simulink model "PID_Dual_Robot"  (R2015b)
settings: Solver=ode4  StartTime=0.0  StopTime=10  FixedStep=0.01  RelTol=1e-3
InitFcn:
  | Set_Parameter_line_circle
StopFcn:
  | DrawResult_Dual
values from neighbouring files (symbols this model uses):
  b = 0.1    [Set_Parameter.m]    (also in Set_Parameter_Single.m; Set_Parameter_line_circle.m; Set_Parameter_line_circle_DC_model_no_vision_controller.m; Set_Parameter_sewing_DC_model_no_vision_controller.m)
  D = [30,30,20,20,20,20,20,20]    [Set_Parameter.m]    (also in Set_Parameter_Single.m; Set_Parameter_line_circle.m; Set_Parameter_line_circle_DC_model_no_vision_controller.m; Set_Parameter_line_circle_no_vision_controller.m = [40,40,40,30,20,30,20,20])
  I = [10,10,5,5,5,2,2,2]    [Set_Parameter.m]    (also in Set_Parameter_Single.m; Set_Parameter_line_circle.m; Set_Parameter_line_circle_DC_model_no_vision_controller.m; Set_Parameter_line_circle_no_vision_controller.m = [5,5,5,2,2,2,1,1])
  IniJointAngle_L = theta_L    [Set_Parameter.m]    (also in Set_Parameter_Single.m; Set_Parameter_line_circle.m; Set_Parameter_line_circle_DC_model_no_vision_controller.m; Set_Parameter_line_circle_no_vision_controller.m)
  IniJointAngle_R = theta_R    [Set_Parameter.m]    (also in Set_Parameter_Single.m; Set_Parameter_line_circle.m; Set_Parameter_line_circle_DC_model_no_vision_controller.m; Set_Parameter_line_circle_no_vision_controller.m)
  J = [0.016,0.016,0.012,0.012,0.01,0.01,0.01]    [Set_Parameter.m]    (also in Set_Parameter_Single.m; Set_Parameter_line_circle.m; Set_Parameter_line_circle_DC_model_no_vision_controller.m; Set_Parameter_line_circle_no_vision_controller.m = [10,10,8,8,4,4,4])
  K = 0.01    [Set_Parameter.m]    (also in Set_Parameter_Single.m; Set_Parameter_line_circle.m; Set_Parameter_line_circle_DC_model_no_vision_controller.m; Set_Parameter_sewing_DC_model_no_vision_controller.m)
  L = 0.5    [Set_Parameter.m]    (also in Set_Parameter_Single.m; Set_Parameter_line_circle.m; Set_Parameter_line_circle_DC_model_no_vision_controller.m; Set_Parameter_sewing_DC_model_no_vision_controller.m)
  P = [60,60,50,50,30,30,20,20]    [Set_Parameter.m]    (also in Set_Parameter_Single.m; Set_Parameter_line_circle.m; Set_Parameter_line_circle_DC_model_no_vision_controller.m = [120,120,100,100,60,60,40,40]; Set_Parameter_line_circle_no_vision_controller.m = [350,100,300,150,50,100,20,20])
  R = R_z1x2y3(PoseAngle(1),PoseAngle(2),PoseAngle(3))    [IK_7DOF_FB7roll.m]    (also in Set_Parameter.m = 1; Set_Parameter_Single.m = 1; Set_Parameter_line_circle.m = 1; Set_Parameter_line_circle_DC_model_no_vision_controller.m = 1)
  TOP_D = 0.9    [Set_Parameter.m]    (also in Set_Parameter_Single.m; Set_Parameter_line_circle.m; Set_Parameter_sewing_DC_model_no_vision_controller.m)
  TOP_I = 1    [Set_Parameter.m]    (also in Set_Parameter_Single.m; Set_Parameter_line_circle.m; Set_Parameter_sewing_DC_model_no_vision_controller.m)
  TOP_P = 5    [Set_Parameter.m]    (also in Set_Parameter_Single.m; Set_Parameter_line_circle.m; Set_Parameter_sewing_DC_model_no_vision_controller.m)
libraries: simulink x14
settings Model: Creator=User  LastModifiedBy=User

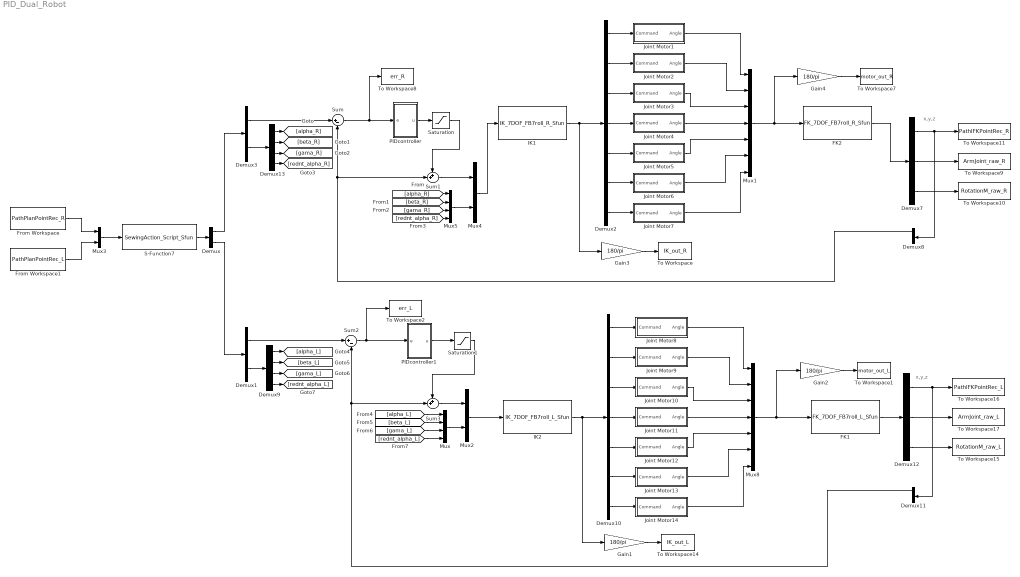
== system PID_Dual_Robot ==
  note: x,y,z
  note: x,y,z
  Demux : Demux  Outputs=[7,7]
  Demux{1,3,8,11} (4 alike) : Demux  Outputs=[3,4]
  Demux10 : Demux  Outputs=7
  Demux12 : Demux  Outputs=[7,30,9]
  Demux13 : Demux
  Demux2 : Demux  Outputs=7
  Demux7 : Demux  Outputs=[7,30,9]
  Demux9 : Demux
  FK1 : S-Function  FunctionName=FK_7DOF_FB7roll_L_Sfun  SFunctionDeploymentMode=off  EnableBusSupport=off
  FK2 : S-Function  FunctionName=FK_7DOF_FB7roll_R_Sfun  SFunctionDeploymentMode=off  EnableBusSupport=off
  From Workspace : FromWorkspace  VariableName=PathPlanPointRec_R  SampleTime=0
  From Workspace1 : FromWorkspace  VariableName=PathPlanPointRec_L  SampleTime=0
  Gain{1..4} (4 alike) : Gain  Gain=180/pi
  IK1 : S-Function  FunctionName=IK_7DOF_FB7roll_R_Sfun  SFunctionDeploymentMode=off  EnableBusSupport=off
  IK2 : S-Function  FunctionName=IK_7DOF_FB7roll_L_Sfun  SFunctionDeploymentMode=off  EnableBusSupport=off
  Joint Motor1 : Subsystem
  Joint Motor10 : Subsystem
  Joint Motor11 : Subsystem
  Joint Motor12 : Subsystem
  Joint Motor13 : Subsystem
  Joint Motor14 : Subsystem
  Joint Motor2 : Subsystem
  Joint Motor3 : Subsystem
  Joint Motor4 : Subsystem
  Joint Motor5 : Subsystem
  Joint Motor6 : Subsystem
  Joint Motor7 : Subsystem
  Joint Motor8 : Subsystem
  Joint Motor9 : Subsystem
  Mux : Mux
  Mux1 : Mux  Inputs=7
  Mux2 : Mux  Inputs=[3,4]
  Mux3 : Mux  Inputs=[7,7]
  Mux4 : Mux  Inputs=[3,4]
  Mux5 : Mux
  Mux8 : Mux  Inputs=7
  PIDcontroller : Subsystem
  PIDcontroller1 : Subsystem
  S-Function7 : S-Function  FunctionName=SewingAction_Script_Sfun  SFunctionDeploymentMode=off  EnableBusSupport=off
  Saturation : Saturate  UpperLimit=50  LowerLimit=-50
  Saturation1 : Saturate  UpperLimit=50  LowerLimit=-50
  Sum : Sum  Inputs=|+-
  Sum1 : Sum  Inputs=++|
  Sum2 : Sum  Inputs=|+-
  Sum3 : Sum  Inputs=++|
  To Workspace : ToWorkspace  VariableName=IK_out_R  SaveFormat=Timeseries  SampleTime=-1
  To Workspace1 : ToWorkspace  VariableName=motor_out_L  SaveFormat=Timeseries  SampleTime=-1
  To Workspace10 : ToWorkspace  VariableName=RotationM_raw_R  SaveFormat=Timeseries  SampleTime=-1
  To Workspace11 : ToWorkspace  VariableName=PathIFKPointRec_R  SaveFormat=Timeseries  SampleTime=-1
  To Workspace14 : ToWorkspace  VariableName=IK_out_L  SaveFormat=Timeseries  SampleTime=-1
  To Workspace15 : ToWorkspace  VariableName=RotationM_raw_L  SaveFormat=Timeseries  SampleTime=-1
  To Workspace16 : ToWorkspace  VariableName=PathIFKPointRec_L  SaveFormat=Timeseries  SampleTime=-1
  To Workspace17 : ToWorkspace  VariableName=ArmJoint_raw_L  SaveFormat=Timeseries  SampleTime=-1
  To Workspace2 : ToWorkspace  VariableName=err_L  SaveFormat=Timeseries  SampleTime=-1
  To Workspace7 : ToWorkspace  VariableName=motor_out_R  SaveFormat=Timeseries  SampleTime=-1
  To Workspace8 : ToWorkspace  VariableName=err_R  SaveFormat=Timeseries  SampleTime=-1
  To Workspace9 : ToWorkspace  VariableName=ArmJoint_raw_R  SaveFormat=Timeseries  SampleTime=-1
  wires:
  Joint Motor3/1(Angle) -> Mux1/3
  Joint Motor1/1(Angle) -> Mux1/1
  Joint Motor2/1(Angle) -> Mux1/2
  Joint Motor4/1(Angle) -> Mux1/4
  Joint Motor5/1(Angle) -> Mux1/5
  Joint Motor6/1(Angle) -> Mux1/6
  Joint Motor7/1(Angle) -> Mux1/7
  Gain3/1 -> To Workspace/1
  Gain4/1 -> To Workspace7/1
  Demux2/6 -> Joint Motor6/1(Command)
  Demux2/5 -> Joint Motor5/1(Command)
  Demux2/4 -> Joint Motor4/1(Command)
  Demux2/1 -> Joint Motor1/1(Command)
  Demux2/2 -> Joint Motor2/1(Command)
  Demux2/3 -> Joint Motor3/1(Command)
  IK1/1 -> Demux2/1, Gain3/1
  Mux1/1 -> Gain4/1, FK2/1
  Sum/1 -> PIDcontroller/1(e), To Workspace8/1
  Mux4/1 -> IK1/1
  PIDcontroller/1(u) -> Saturation/1
  Saturation/1 -> Sum1/1
  FK2/1 -> Demux7/1
  Demux7/1 -> To Workspace11/1, Demux8/1
  Demux7/2 -> To Workspace9/1
  Demux7/3 -> To Workspace10/1
  Demux8/1 -> Sum/2, Sum1/2
  S-Function7/1 -> Demux/1
  Demux/1 -> Demux3/1
  Demux/2 -> Demux1/1
  Sum2/1 -> To Workspace2/1, PIDcontroller1/1(e)
  PIDcontroller1/1(u) -> Saturation1/1
  Saturation1/1 -> Sum3/1
  Demux9/1 -> [alpha_L]
  Demux9/2 -> [beta_L]
  Demux9/3 -> [gama_L]
  Demux9/4 -> [rednt_alpha_L]
  Demux1/2 -> Demux9/1
  [alpha_L] -> Mux/1
  [beta_L] -> Mux/2
  [gama_L] -> Mux/3
  [rednt_alpha_L] -> Mux/4
  Mux/1 -> Mux2/2
  Joint Motor10/1(Angle) -> Mux8/3
  Joint Motor8/1(Angle) -> Mux8/1
  Joint Motor9/1(Angle) -> Mux8/2
  Joint Motor11/1(Angle) -> Mux8/4
  Joint Motor12/1(Angle) -> Mux8/5
  Joint Motor13/1(Angle) -> Mux8/6
  Joint Motor14/1(Angle) -> Mux8/7
  Demux10/7 -> Joint Motor14/1(Command)
  Demux10/6 -> Joint Motor13/1(Command)
  Demux10/5 -> Joint Motor12/1(Command)
  Demux10/4 -> Joint Motor11/1(Command)
  Demux10/1 -> Joint Motor8/1(Command)
  Demux10/2 -> Joint Motor9/1(Command)
  Demux10/3 -> Joint Motor10/1(Command)
  Gain1/1 -> To Workspace14/1
  IK2/1 -> Demux10/1, Gain1/1
  FK1/1 -> Demux12/1
  Demux12/2 -> To Workspace17/1
  Demux12/1 -> To Workspace16/1, Demux11/1
  Demux12/3 -> To Workspace15/1
  Demux3/1 -> Sum/1
  Demux3/2 -> Demux13/1
  Demux13/2 -> [beta_R]
  Demux13/3 -> [gama_R]
  Demux13/4 -> [rednt_alpha_R]
  Gain2/1 -> To Workspace1/1
  Mux8/1 -> FK1/1, Gain2/1
  Mux3/1 -> S-Function7/1
  From Workspace/1 -> Mux3/1
  From Workspace1/1 -> Mux3/2
  Mux2/1 -> IK2/1
  Demux1/1 -> Sum2/1
  Sum3/1 -> Mux2/1
  Demux11/1 -> Sum3/2, Sum2/2
  Sum1/1 -> Mux4/1
  Mux5/1 -> Mux4/2
  [alpha_R] -> Mux5/1
  [beta_R] -> Mux5/2
  [gama_R] -> Mux5/3
  [rednt_alpha_R] -> Mux5/4
  Demux2/7 -> Joint Motor7/1(Command)
  Demux13/1 -> [alpha_R]

== system PID_Dual_Robot/Joint Motor1 ==
  Command : Inport
  Constant : Constant  Value=IniJointAngle_R(1)
  DC motor : Subsystem
  Gain : Gain  Gain=2
  Integrator : Integrator  InitialConditionSource=external
  PID Controller : simulink/Continuous/PID Controller  Controller=PID  TimeDomain=Continuous-time  SampleTime=-1  IntegratorMethod=Forward Euler  FilterMethod=Forward Euler  Form=Parallel  UseFilter=on  ControllerParametersSource=internal  P=P(1)  I=I(1)  D=D(1)  N=0  InitialConditionSource=internal  InitialConditionForIntegrator=0  InitialConditionForFilter=0  ExternalReset=none  LimitOutput=off  UpperSaturationLimit=inf  LowerSaturationLimit=-inf  LinearizeAsGain=on  AntiWindupMode=none  Kb=1  TrackingMode=off  Kt=1  PParamMin=[]  PParamMax=[]  IParamMin=[]  IParamMax=[]  DParamMin=[]  DParamMax=[]  NParamMin=[]  NParamMax=[]  KbParamMin=[]  KbParamMax=[]  KtParamMin=[]  KtParamMax=[]  POutMin=[]  POutMax=[]  IOutMin=[]  IOutMax=[]  DOutMin=[]  DOutMax=[]  NOutMin=[]  NOutMax=[]  KbOutMin=[]  KbOutMax=[]  KtOutMin=[]  KtOutMax=[]  IntegratorOutMin=[]  IntegratorOutMax=[]  FilterOutMin=[]  FilterOutMax=[]  SumOutMin=[]  SumOutMax=[]  SumI1OutMin=[]  SumI1OutMax=[]  SumI2OutMin=[]  SumI2OutMax=[]  SumI3OutMin=[]  SumI3OutMax=[]  SumDOutMin=[]  SumDOutMax=[]  SaturationOutMin=[]  SaturationOutMax=[]  IntegratorContinuousStateAttributes=''  IntegratorStateMustResolveToSignalObject=off  IntegratorRTWStateStorageClass=Auto  FilterContinuousStateAttributes=''  FilterStateMustResolveToSignalObject=off  FilterRTWStateStorageClass=Auto  DifferentiatorICPrevScaledInput=0  DifferentiatorOutMin=[]  DifferentiatorOutMax=[]
  Sum : Sum  Inputs=|+-
  Sum1 : Sum  Inputs=|+-
  Angle : Outport
  wires:
  Sum/1 -> PID Controller/1
  PID Controller/1 -> DC motor/1(Voltage)
  DC motor/1(Speed) -> Sum/2, Integrator/1
  Integrator/1 -> Angle/1, Sum1/2
  Command/1 -> Sum1/1
  Sum1/1 -> Gain/1
  Gain/1 -> Sum/1
  Constant/1 -> Integrator/2

== system PID_Dual_Robot/Joint Motor10 ==
  Command : Inport
  Constant : Constant  Value=IniJointAngle_L(3)
  DC motor : Subsystem
  Gain : Gain  Gain=2
  Integrator : Integrator  InitialConditionSource=external
  PID Controller : simulink/Continuous/PID Controller  Controller=PID  TimeDomain=Continuous-time  SampleTime=-1  IntegratorMethod=Forward Euler  FilterMethod=Forward Euler  Form=Parallel  UseFilter=on  ControllerParametersSource=internal  P=P(3)  I=I(3)  D=D(3)  N=0  InitialConditionSource=internal  InitialConditionForIntegrator=0  InitialConditionForFilter=0  ExternalReset=none  LimitOutput=off  UpperSaturationLimit=inf  LowerSaturationLimit=-inf  LinearizeAsGain=on  AntiWindupMode=none  Kb=1  TrackingMode=off  Kt=1  PParamMin=[]  PParamMax=[]  IParamMin=[]  IParamMax=[]  DParamMin=[]  DParamMax=[]  NParamMin=[]  NParamMax=[]  KbParamMin=[]  KbParamMax=[]  KtParamMin=[]  KtParamMax=[]  POutMin=[]  POutMax=[]  IOutMin=[]  IOutMax=[]  DOutMin=[]  DOutMax=[]  NOutMin=[]  NOutMax=[]  KbOutMin=[]  KbOutMax=[]  KtOutMin=[]  KtOutMax=[]  IntegratorOutMin=[]  IntegratorOutMax=[]  FilterOutMin=[]  FilterOutMax=[]  SumOutMin=[]  SumOutMax=[]  SumI1OutMin=[]  SumI1OutMax=[]  SumI2OutMin=[]  SumI2OutMax=[]  SumI3OutMin=[]  SumI3OutMax=[]  SumDOutMin=[]  SumDOutMax=[]  SaturationOutMin=[]  SaturationOutMax=[]  IntegratorContinuousStateAttributes=''  IntegratorStateMustResolveToSignalObject=off  IntegratorRTWStateStorageClass=Auto  FilterContinuousStateAttributes=''  FilterStateMustResolveToSignalObject=off  FilterRTWStateStorageClass=Auto  DifferentiatorICPrevScaledInput=0  DifferentiatorOutMin=[]  DifferentiatorOutMax=[]
  Sum : Sum  Inputs=|+-
  Sum1 : Sum  Inputs=|+-
  Angle : Outport
  wires:
  Sum/1 -> PID Controller/1
  PID Controller/1 -> DC motor/1(Voltage)
  DC motor/1(Speed) -> Sum/2, Integrator/1
  Integrator/1 -> Angle/1, Sum1/2
  Command/1 -> Sum1/1
  Sum1/1 -> Gain/1
  Gain/1 -> Sum/1
  Constant/1 -> Integrator/2

== system PID_Dual_Robot/Joint Motor11 ==
  Command : Inport
  Constant : Constant  Value=IniJointAngle_L(4)
  DC motor : Subsystem
  Gain : Gain  Gain=2
  Integrator : Integrator  InitialConditionSource=external
  PID Controller : simulink/Continuous/PID Controller  Controller=PID  TimeDomain=Continuous-time  SampleTime=-1  IntegratorMethod=Forward Euler  FilterMethod=Forward Euler  Form=Parallel  UseFilter=on  ControllerParametersSource=internal  P=P(4)  I=I(4)  D=D(4)  N=0  InitialConditionSource=internal  InitialConditionForIntegrator=0  InitialConditionForFilter=0  ExternalReset=none  LimitOutput=off  UpperSaturationLimit=inf  LowerSaturationLimit=-inf  LinearizeAsGain=on  AntiWindupMode=none  Kb=1  TrackingMode=off  Kt=1  PParamMin=[]  PParamMax=[]  IParamMin=[]  IParamMax=[]  DParamMin=[]  DParamMax=[]  NParamMin=[]  NParamMax=[]  KbParamMin=[]  KbParamMax=[]  KtParamMin=[]  KtParamMax=[]  POutMin=[]  POutMax=[]  IOutMin=[]  IOutMax=[]  DOutMin=[]  DOutMax=[]  NOutMin=[]  NOutMax=[]  KbOutMin=[]  KbOutMax=[]  KtOutMin=[]  KtOutMax=[]  IntegratorOutMin=[]  IntegratorOutMax=[]  FilterOutMin=[]  FilterOutMax=[]  SumOutMin=[]  SumOutMax=[]  SumI1OutMin=[]  SumI1OutMax=[]  SumI2OutMin=[]  SumI2OutMax=[]  SumI3OutMin=[]  SumI3OutMax=[]  SumDOutMin=[]  SumDOutMax=[]  SaturationOutMin=[]  SaturationOutMax=[]  IntegratorContinuousStateAttributes=''  IntegratorStateMustResolveToSignalObject=off  IntegratorRTWStateStorageClass=Auto  FilterContinuousStateAttributes=''  FilterStateMustResolveToSignalObject=off  FilterRTWStateStorageClass=Auto  DifferentiatorICPrevScaledInput=0  DifferentiatorOutMin=[]  DifferentiatorOutMax=[]
  Sum : Sum  Inputs=|+-
  Sum1 : Sum  Inputs=|+-
  Angle : Outport
  wires:
  Sum/1 -> PID Controller/1
  PID Controller/1 -> DC motor/1(Voltage)
  DC motor/1(Speed) -> Sum/2, Integrator/1
  Integrator/1 -> Angle/1, Sum1/2
  Command/1 -> Sum1/1
  Sum1/1 -> Gain/1
  Gain/1 -> Sum/1
  Constant/1 -> Integrator/2

== system PID_Dual_Robot/Joint Motor12 ==
  Command : Inport
  Constant : Constant  Value=IniJointAngle_L(5)
  DC motor : Subsystem
  Gain : Gain  Gain=2
  Integrator : Integrator  InitialConditionSource=external
  PID Controller : simulink/Continuous/PID Controller  Controller=PID  TimeDomain=Continuous-time  SampleTime=-1  IntegratorMethod=Forward Euler  FilterMethod=Forward Euler  Form=Parallel  UseFilter=on  ControllerParametersSource=internal  P=P(5)  I=I(5)  D=D(5)  N=0  InitialConditionSource=internal  InitialConditionForIntegrator=0  InitialConditionForFilter=0  ExternalReset=none  LimitOutput=off  UpperSaturationLimit=inf  LowerSaturationLimit=-inf  LinearizeAsGain=on  AntiWindupMode=none  Kb=1  TrackingMode=off  Kt=1  PParamMin=[]  PParamMax=[]  IParamMin=[]  IParamMax=[]  DParamMin=[]  DParamMax=[]  NParamMin=[]  NParamMax=[]  KbParamMin=[]  KbParamMax=[]  KtParamMin=[]  KtParamMax=[]  POutMin=[]  POutMax=[]  IOutMin=[]  IOutMax=[]  DOutMin=[]  DOutMax=[]  NOutMin=[]  NOutMax=[]  KbOutMin=[]  KbOutMax=[]  KtOutMin=[]  KtOutMax=[]  IntegratorOutMin=[]  IntegratorOutMax=[]  FilterOutMin=[]  FilterOutMax=[]  SumOutMin=[]  SumOutMax=[]  SumI1OutMin=[]  SumI1OutMax=[]  SumI2OutMin=[]  SumI2OutMax=[]  SumI3OutMin=[]  SumI3OutMax=[]  SumDOutMin=[]  SumDOutMax=[]  SaturationOutMin=[]  SaturationOutMax=[]  IntegratorContinuousStateAttributes=''  IntegratorStateMustResolveToSignalObject=off  IntegratorRTWStateStorageClass=Auto  FilterContinuousStateAttributes=''  FilterStateMustResolveToSignalObject=off  FilterRTWStateStorageClass=Auto  DifferentiatorICPrevScaledInput=0  DifferentiatorOutMin=[]  DifferentiatorOutMax=[]
  Sum : Sum  Inputs=|+-
  Sum1 : Sum  Inputs=|+-
  Angle : Outport
  wires:
  Sum/1 -> PID Controller/1
  PID Controller/1 -> DC motor/1(Voltage)
  DC motor/1(Speed) -> Sum/2, Integrator/1
  Integrator/1 -> Angle/1, Sum1/2
  Command/1 -> Sum1/1
  Sum1/1 -> Gain/1
  Gain/1 -> Sum/1
  Constant/1 -> Integrator/2

== system PID_Dual_Robot/Joint Motor13 ==
  Command : Inport
  Constant : Constant  Value=IniJointAngle_L(6)
  DC motor : Subsystem
  Gain : Gain  Gain=2
  Integrator : Integrator  InitialConditionSource=external
  PID Controller : simulink/Continuous/PID Controller  Controller=PID  TimeDomain=Continuous-time  SampleTime=-1  IntegratorMethod=Forward Euler  FilterMethod=Forward Euler  Form=Parallel  UseFilter=on  ControllerParametersSource=internal  P=P(6)  I=I(6)  D=D(6)  N=0  InitialConditionSource=internal  InitialConditionForIntegrator=0  InitialConditionForFilter=0  ExternalReset=none  LimitOutput=off  UpperSaturationLimit=inf  LowerSaturationLimit=-inf  LinearizeAsGain=on  AntiWindupMode=none  Kb=1  TrackingMode=off  Kt=1  PParamMin=[]  PParamMax=[]  IParamMin=[]  IParamMax=[]  DParamMin=[]  DParamMax=[]  NParamMin=[]  NParamMax=[]  KbParamMin=[]  KbParamMax=[]  KtParamMin=[]  KtParamMax=[]  POutMin=[]  POutMax=[]  IOutMin=[]  IOutMax=[]  DOutMin=[]  DOutMax=[]  NOutMin=[]  NOutMax=[]  KbOutMin=[]  KbOutMax=[]  KtOutMin=[]  KtOutMax=[]  IntegratorOutMin=[]  IntegratorOutMax=[]  FilterOutMin=[]  FilterOutMax=[]  SumOutMin=[]  SumOutMax=[]  SumI1OutMin=[]  SumI1OutMax=[]  SumI2OutMin=[]  SumI2OutMax=[]  SumI3OutMin=[]  SumI3OutMax=[]  SumDOutMin=[]  SumDOutMax=[]  SaturationOutMin=[]  SaturationOutMax=[]  IntegratorContinuousStateAttributes=''  IntegratorStateMustResolveToSignalObject=off  IntegratorRTWStateStorageClass=Auto  FilterContinuousStateAttributes=''  FilterStateMustResolveToSignalObject=off  FilterRTWStateStorageClass=Auto  DifferentiatorICPrevScaledInput=0  DifferentiatorOutMin=[]  DifferentiatorOutMax=[]
  Sum : Sum  Inputs=|+-
  Sum1 : Sum  Inputs=|+-
  Angle : Outport
  wires:
  Sum/1 -> PID Controller/1
  PID Controller/1 -> DC motor/1(Voltage)
  DC motor/1(Speed) -> Sum/2, Integrator/1
  Integrator/1 -> Angle/1, Sum1/2
  Command/1 -> Sum1/1
  Sum1/1 -> Gain/1
  Gain/1 -> Sum/1
  Constant/1 -> Integrator/2

== system PID_Dual_Robot/Joint Motor14 ==
  Command : Inport
  Constant : Constant  Value=IniJointAngle_L(7)
  DC motor : Subsystem
  Gain : Gain  Gain=2
  Integrator : Integrator  InitialConditionSource=external
  PID Controller : simulink/Continuous/PID Controller  Controller=PID  TimeDomain=Continuous-time  SampleTime=-1  IntegratorMethod=Forward Euler  FilterMethod=Forward Euler  Form=Parallel  UseFilter=on  ControllerParametersSource=internal  P=P(7)  I=I(7)  D=D(7)  N=0  InitialConditionSource=internal  InitialConditionForIntegrator=0  InitialConditionForFilter=0  ExternalReset=none  LimitOutput=off  UpperSaturationLimit=inf  LowerSaturationLimit=-inf  LinearizeAsGain=on  AntiWindupMode=none  Kb=1  TrackingMode=off  Kt=1  PParamMin=[]  PParamMax=[]  IParamMin=[]  IParamMax=[]  DParamMin=[]  DParamMax=[]  NParamMin=[]  NParamMax=[]  KbParamMin=[]  KbParamMax=[]  KtParamMin=[]  KtParamMax=[]  POutMin=[]  POutMax=[]  IOutMin=[]  IOutMax=[]  DOutMin=[]  DOutMax=[]  NOutMin=[]  NOutMax=[]  KbOutMin=[]  KbOutMax=[]  KtOutMin=[]  KtOutMax=[]  IntegratorOutMin=[]  IntegratorOutMax=[]  FilterOutMin=[]  FilterOutMax=[]  SumOutMin=[]  SumOutMax=[]  SumI1OutMin=[]  SumI1OutMax=[]  SumI2OutMin=[]  SumI2OutMax=[]  SumI3OutMin=[]  SumI3OutMax=[]  SumDOutMin=[]  SumDOutMax=[]  SaturationOutMin=[]  SaturationOutMax=[]  IntegratorContinuousStateAttributes=''  IntegratorStateMustResolveToSignalObject=off  IntegratorRTWStateStorageClass=Auto  FilterContinuousStateAttributes=''  FilterStateMustResolveToSignalObject=off  FilterRTWStateStorageClass=Auto  DifferentiatorICPrevScaledInput=0  DifferentiatorOutMin=[]  DifferentiatorOutMax=[]
  Sum : Sum  Inputs=|+-
  Sum1 : Sum  Inputs=|+-
  Angle : Outport
  wires:
  Sum/1 -> PID Controller/1
  PID Controller/1 -> DC motor/1(Voltage)
  DC motor/1(Speed) -> Sum/2, Integrator/1
  Integrator/1 -> Angle/1, Sum1/2
  Command/1 -> Sum1/1
  Sum1/1 -> Gain/1
  Gain/1 -> Sum/1
  Constant/1 -> Integrator/2

== system PID_Dual_Robot/Joint Motor2 ==
  Command : Inport
  Constant : Constant  Value=IniJointAngle_R(2)
  DC motor : Subsystem
  Gain : Gain  Gain=2
  Integrator : Integrator  InitialConditionSource=external
  PID Controller : simulink/Continuous/PID Controller  Controller=PID  TimeDomain=Continuous-time  SampleTime=-1  IntegratorMethod=Forward Euler  FilterMethod=Forward Euler  Form=Parallel  UseFilter=on  ControllerParametersSource=internal  P=P(2)  I=I(2)  D=D(2)  N=0  InitialConditionSource=internal  InitialConditionForIntegrator=0  InitialConditionForFilter=0  ExternalReset=none  LimitOutput=off  UpperSaturationLimit=inf  LowerSaturationLimit=-inf  LinearizeAsGain=on  AntiWindupMode=none  Kb=1  TrackingMode=off  Kt=1  PParamMin=[]  PParamMax=[]  IParamMin=[]  IParamMax=[]  DParamMin=[]  DParamMax=[]  NParamMin=[]  NParamMax=[]  KbParamMin=[]  KbParamMax=[]  KtParamMin=[]  KtParamMax=[]  POutMin=[]  POutMax=[]  IOutMin=[]  IOutMax=[]  DOutMin=[]  DOutMax=[]  NOutMin=[]  NOutMax=[]  KbOutMin=[]  KbOutMax=[]  KtOutMin=[]  KtOutMax=[]  IntegratorOutMin=[]  IntegratorOutMax=[]  FilterOutMin=[]  FilterOutMax=[]  SumOutMin=[]  SumOutMax=[]  SumI1OutMin=[]  SumI1OutMax=[]  SumI2OutMin=[]  SumI2OutMax=[]  SumI3OutMin=[]  SumI3OutMax=[]  SumDOutMin=[]  SumDOutMax=[]  SaturationOutMin=[]  SaturationOutMax=[]  IntegratorContinuousStateAttributes=''  IntegratorStateMustResolveToSignalObject=off  IntegratorRTWStateStorageClass=Auto  FilterContinuousStateAttributes=''  FilterStateMustResolveToSignalObject=off  FilterRTWStateStorageClass=Auto  DifferentiatorICPrevScaledInput=0  DifferentiatorOutMin=[]  DifferentiatorOutMax=[]
  Sum : Sum  Inputs=|+-
  Sum1 : Sum  Inputs=|+-
  Angle : Outport
  wires:
  Sum/1 -> PID Controller/1
  PID Controller/1 -> DC motor/1(Voltage)
  DC motor/1(Speed) -> Sum/2, Integrator/1
  Integrator/1 -> Angle/1, Sum1/2
  Command/1 -> Sum1/1
  Sum1/1 -> Gain/1
  Gain/1 -> Sum/1
  Constant/1 -> Integrator/2

== system PID_Dual_Robot/Joint Motor3 ==
  Command : Inport
  Constant : Constant  Value=IniJointAngle_R(3)
  DC motor : Subsystem
  Gain : Gain  Gain=2
  Integrator : Integrator  InitialConditionSource=external
  PID Controller : simulink/Continuous/PID Controller  Controller=PID  TimeDomain=Continuous-time  SampleTime=-1  IntegratorMethod=Forward Euler  FilterMethod=Forward Euler  Form=Parallel  UseFilter=on  ControllerParametersSource=internal  P=P(3)  I=I(3)  D=D(3)  N=0  InitialConditionSource=internal  InitialConditionForIntegrator=0  InitialConditionForFilter=0  ExternalReset=none  LimitOutput=off  UpperSaturationLimit=inf  LowerSaturationLimit=-inf  LinearizeAsGain=on  AntiWindupMode=none  Kb=1  TrackingMode=off  Kt=1  PParamMin=[]  PParamMax=[]  IParamMin=[]  IParamMax=[]  DParamMin=[]  DParamMax=[]  NParamMin=[]  NParamMax=[]  KbParamMin=[]  KbParamMax=[]  KtParamMin=[]  KtParamMax=[]  POutMin=[]  POutMax=[]  IOutMin=[]  IOutMax=[]  DOutMin=[]  DOutMax=[]  NOutMin=[]  NOutMax=[]  KbOutMin=[]  KbOutMax=[]  KtOutMin=[]  KtOutMax=[]  IntegratorOutMin=[]  IntegratorOutMax=[]  FilterOutMin=[]  FilterOutMax=[]  SumOutMin=[]  SumOutMax=[]  SumI1OutMin=[]  SumI1OutMax=[]  SumI2OutMin=[]  SumI2OutMax=[]  SumI3OutMin=[]  SumI3OutMax=[]  SumDOutMin=[]  SumDOutMax=[]  SaturationOutMin=[]  SaturationOutMax=[]  IntegratorContinuousStateAttributes=''  IntegratorStateMustResolveToSignalObject=off  IntegratorRTWStateStorageClass=Auto  FilterContinuousStateAttributes=''  FilterStateMustResolveToSignalObject=off  FilterRTWStateStorageClass=Auto  DifferentiatorICPrevScaledInput=0  DifferentiatorOutMin=[]  DifferentiatorOutMax=[]
  Sum : Sum  Inputs=|+-
  Sum1 : Sum  Inputs=|+-
  Angle : Outport
  wires:
  Sum/1 -> PID Controller/1
  PID Controller/1 -> DC motor/1(Voltage)
  DC motor/1(Speed) -> Sum/2, Integrator/1
  Integrator/1 -> Angle/1, Sum1/2
  Command/1 -> Sum1/1
  Sum1/1 -> Gain/1
  Gain/1 -> Sum/1
  Constant/1 -> Integrator/2

== system PID_Dual_Robot/Joint Motor4 ==
  Command : Inport
  Constant : Constant  Value=IniJointAngle_R(4)
  DC motor : Subsystem
  Gain : Gain  Gain=2
  Integrator : Integrator  InitialConditionSource=external
  PID Controller : simulink/Continuous/PID Controller  Controller=PID  TimeDomain=Continuous-time  SampleTime=-1  IntegratorMethod=Forward Euler  FilterMethod=Forward Euler  Form=Parallel  UseFilter=on  ControllerParametersSource=internal  P=P(4)  I=I(4)  D=D(4)  N=0  InitialConditionSource=internal  InitialConditionForIntegrator=0  InitialConditionForFilter=0  ExternalReset=none  LimitOutput=off  UpperSaturationLimit=inf  LowerSaturationLimit=-inf  LinearizeAsGain=on  AntiWindupMode=none  Kb=1  TrackingMode=off  Kt=1  PParamMin=[]  PParamMax=[]  IParamMin=[]  IParamMax=[]  DParamMin=[]  DParamMax=[]  NParamMin=[]  NParamMax=[]  KbParamMin=[]  KbParamMax=[]  KtParamMin=[]  KtParamMax=[]  POutMin=[]  POutMax=[]  IOutMin=[]  IOutMax=[]  DOutMin=[]  DOutMax=[]  NOutMin=[]  NOutMax=[]  KbOutMin=[]  KbOutMax=[]  KtOutMin=[]  KtOutMax=[]  IntegratorOutMin=[]  IntegratorOutMax=[]  FilterOutMin=[]  FilterOutMax=[]  SumOutMin=[]  SumOutMax=[]  SumI1OutMin=[]  SumI1OutMax=[]  SumI2OutMin=[]  SumI2OutMax=[]  SumI3OutMin=[]  SumI3OutMax=[]  SumDOutMin=[]  SumDOutMax=[]  SaturationOutMin=[]  SaturationOutMax=[]  IntegratorContinuousStateAttributes=''  IntegratorStateMustResolveToSignalObject=off  IntegratorRTWStateStorageClass=Auto  FilterContinuousStateAttributes=''  FilterStateMustResolveToSignalObject=off  FilterRTWStateStorageClass=Auto  DifferentiatorICPrevScaledInput=0  DifferentiatorOutMin=[]  DifferentiatorOutMax=[]
  Sum : Sum  Inputs=|+-
  Sum1 : Sum  Inputs=|+-
  Angle : Outport
  wires:
  Sum/1 -> PID Controller/1
  PID Controller/1 -> DC motor/1(Voltage)
  DC motor/1(Speed) -> Sum/2, Integrator/1
  Integrator/1 -> Angle/1, Sum1/2
  Command/1 -> Sum1/1
  Sum1/1 -> Gain/1
  Gain/1 -> Sum/1
  Constant/1 -> Integrator/2

== system PID_Dual_Robot/Joint Motor5 ==
  Command : Inport
  Constant : Constant  Value=IniJointAngle_R(5)
  DC motor : Subsystem
  Gain : Gain  Gain=2
  Integrator : Integrator  InitialConditionSource=external
  PID Controller : simulink/Continuous/PID Controller  Controller=PID  TimeDomain=Continuous-time  SampleTime=-1  IntegratorMethod=Forward Euler  FilterMethod=Forward Euler  Form=Parallel  UseFilter=on  ControllerParametersSource=internal  P=P(5)  I=I(5)  D=D(5)  N=0  InitialConditionSource=internal  InitialConditionForIntegrator=0  InitialConditionForFilter=0  ExternalReset=none  LimitOutput=off  UpperSaturationLimit=inf  LowerSaturationLimit=-inf  LinearizeAsGain=on  AntiWindupMode=none  Kb=1  TrackingMode=off  Kt=1  PParamMin=[]  PParamMax=[]  IParamMin=[]  IParamMax=[]  DParamMin=[]  DParamMax=[]  NParamMin=[]  NParamMax=[]  KbParamMin=[]  KbParamMax=[]  KtParamMin=[]  KtParamMax=[]  POutMin=[]  POutMax=[]  IOutMin=[]  IOutMax=[]  DOutMin=[]  DOutMax=[]  NOutMin=[]  NOutMax=[]  KbOutMin=[]  KbOutMax=[]  KtOutMin=[]  KtOutMax=[]  IntegratorOutMin=[]  IntegratorOutMax=[]  FilterOutMin=[]  FilterOutMax=[]  SumOutMin=[]  SumOutMax=[]  SumI1OutMin=[]  SumI1OutMax=[]  SumI2OutMin=[]  SumI2OutMax=[]  SumI3OutMin=[]  SumI3OutMax=[]  SumDOutMin=[]  SumDOutMax=[]  SaturationOutMin=[]  SaturationOutMax=[]  IntegratorContinuousStateAttributes=''  IntegratorStateMustResolveToSignalObject=off  IntegratorRTWStateStorageClass=Auto  FilterContinuousStateAttributes=''  FilterStateMustResolveToSignalObject=off  FilterRTWStateStorageClass=Auto  DifferentiatorICPrevScaledInput=0  DifferentiatorOutMin=[]  DifferentiatorOutMax=[]
  Sum : Sum  Inputs=|+-
  Sum1 : Sum  Inputs=|+-
  Angle : Outport
  wires:
  Sum/1 -> PID Controller/1
  PID Controller/1 -> DC motor/1(Voltage)
  DC motor/1(Speed) -> Sum/2, Integrator/1
  Integrator/1 -> Angle/1, Sum1/2
  Command/1 -> Sum1/1
  Sum1/1 -> Gain/1
  Gain/1 -> Sum/1
  Constant/1 -> Integrator/2

== system PID_Dual_Robot/Joint Motor6 ==
  Command : Inport
  Constant : Constant  Value=IniJointAngle_R(6)
  DC motor : Subsystem
  Gain : Gain  Gain=2
  Integrator : Integrator  InitialConditionSource=external
  PID Controller : simulink/Continuous/PID Controller  Controller=PID  TimeDomain=Continuous-time  SampleTime=-1  IntegratorMethod=Forward Euler  FilterMethod=Forward Euler  Form=Parallel  UseFilter=on  ControllerParametersSource=internal  P=P(6)  I=I(6)  D=D(6)  N=0  InitialConditionSource=internal  InitialConditionForIntegrator=0  InitialConditionForFilter=0  ExternalReset=none  LimitOutput=off  UpperSaturationLimit=inf  LowerSaturationLimit=-inf  LinearizeAsGain=on  AntiWindupMode=none  Kb=1  TrackingMode=off  Kt=1  PParamMin=[]  PParamMax=[]  IParamMin=[]  IParamMax=[]  DParamMin=[]  DParamMax=[]  NParamMin=[]  NParamMax=[]  KbParamMin=[]  KbParamMax=[]  KtParamMin=[]  KtParamMax=[]  POutMin=[]  POutMax=[]  IOutMin=[]  IOutMax=[]  DOutMin=[]  DOutMax=[]  NOutMin=[]  NOutMax=[]  KbOutMin=[]  KbOutMax=[]  KtOutMin=[]  KtOutMax=[]  IntegratorOutMin=[]  IntegratorOutMax=[]  FilterOutMin=[]  FilterOutMax=[]  SumOutMin=[]  SumOutMax=[]  SumI1OutMin=[]  SumI1OutMax=[]  SumI2OutMin=[]  SumI2OutMax=[]  SumI3OutMin=[]  SumI3OutMax=[]  SumDOutMin=[]  SumDOutMax=[]  SaturationOutMin=[]  SaturationOutMax=[]  IntegratorContinuousStateAttributes=''  IntegratorStateMustResolveToSignalObject=off  IntegratorRTWStateStorageClass=Auto  FilterContinuousStateAttributes=''  FilterStateMustResolveToSignalObject=off  FilterRTWStateStorageClass=Auto  DifferentiatorICPrevScaledInput=0  DifferentiatorOutMin=[]  DifferentiatorOutMax=[]
  Sum : Sum  Inputs=|+-
  Sum1 : Sum  Inputs=|+-
  Angle : Outport
  wires:
  Sum/1 -> PID Controller/1
  PID Controller/1 -> DC motor/1(Voltage)
  DC motor/1(Speed) -> Sum/2, Integrator/1
  Integrator/1 -> Angle/1, Sum1/2
  Command/1 -> Sum1/1
  Sum1/1 -> Gain/1
  Gain/1 -> Sum/1
  Constant/1 -> Integrator/2

== system PID_Dual_Robot/Joint Motor7 ==
  Command : Inport
  Constant : Constant  Value=IniJointAngle_R(7)
  DC motor : Subsystem
  Gain : Gain  Gain=2
  Integrator : Integrator  InitialConditionSource=external
  PID Controller : simulink/Continuous/PID Controller  Controller=PID  TimeDomain=Continuous-time  SampleTime=-1  IntegratorMethod=Forward Euler  FilterMethod=Forward Euler  Form=Parallel  UseFilter=on  ControllerParametersSource=internal  P=P(7)  I=I(7)  D=D(7)  N=0  InitialConditionSource=internal  InitialConditionForIntegrator=0  InitialConditionForFilter=0  ExternalReset=none  LimitOutput=off  UpperSaturationLimit=inf  LowerSaturationLimit=-inf  LinearizeAsGain=on  AntiWindupMode=none  Kb=1  TrackingMode=off  Kt=1  PParamMin=[]  PParamMax=[]  IParamMin=[]  IParamMax=[]  DParamMin=[]  DParamMax=[]  NParamMin=[]  NParamMax=[]  KbParamMin=[]  KbParamMax=[]  KtParamMin=[]  KtParamMax=[]  POutMin=[]  POutMax=[]  IOutMin=[]  IOutMax=[]  DOutMin=[]  DOutMax=[]  NOutMin=[]  NOutMax=[]  KbOutMin=[]  KbOutMax=[]  KtOutMin=[]  KtOutMax=[]  IntegratorOutMin=[]  IntegratorOutMax=[]  FilterOutMin=[]  FilterOutMax=[]  SumOutMin=[]  SumOutMax=[]  SumI1OutMin=[]  SumI1OutMax=[]  SumI2OutMin=[]  SumI2OutMax=[]  SumI3OutMin=[]  SumI3OutMax=[]  SumDOutMin=[]  SumDOutMax=[]  SaturationOutMin=[]  SaturationOutMax=[]  IntegratorContinuousStateAttributes=''  IntegratorStateMustResolveToSignalObject=off  IntegratorRTWStateStorageClass=Auto  FilterContinuousStateAttributes=''  FilterStateMustResolveToSignalObject=off  FilterRTWStateStorageClass=Auto  DifferentiatorICPrevScaledInput=0  DifferentiatorOutMin=[]  DifferentiatorOutMax=[]
  Sum : Sum  Inputs=|+-
  Sum1 : Sum  Inputs=|+-
  Angle : Outport
  wires:
  Sum/1 -> PID Controller/1
  PID Controller/1 -> DC motor/1(Voltage)
  DC motor/1(Speed) -> Sum/2, Integrator/1
  Integrator/1 -> Angle/1, Sum1/2
  Command/1 -> Sum1/1
  Sum1/1 -> Gain/1
  Gain/1 -> Sum/1
  Constant/1 -> Integrator/2

== system PID_Dual_Robot/Joint Motor8 ==
  Command : Inport
  Constant : Constant  Value=IniJointAngle_L(1)
  DC motor : Subsystem
  Gain : Gain  Gain=2
  Integrator : Integrator  InitialConditionSource=external
  PID Controller : simulink/Continuous/PID Controller  Controller=PID  TimeDomain=Continuous-time  SampleTime=-1  IntegratorMethod=Forward Euler  FilterMethod=Forward Euler  Form=Parallel  UseFilter=on  ControllerParametersSource=internal  P=P(1)  I=I(1)  D=D(1)  N=0  InitialConditionSource=internal  InitialConditionForIntegrator=0  InitialConditionForFilter=0  ExternalReset=none  LimitOutput=off  UpperSaturationLimit=inf  LowerSaturationLimit=-inf  LinearizeAsGain=on  AntiWindupMode=none  Kb=1  TrackingMode=off  Kt=1  PParamMin=[]  PParamMax=[]  IParamMin=[]  IParamMax=[]  DParamMin=[]  DParamMax=[]  NParamMin=[]  NParamMax=[]  KbParamMin=[]  KbParamMax=[]  KtParamMin=[]  KtParamMax=[]  POutMin=[]  POutMax=[]  IOutMin=[]  IOutMax=[]  DOutMin=[]  DOutMax=[]  NOutMin=[]  NOutMax=[]  KbOutMin=[]  KbOutMax=[]  KtOutMin=[]  KtOutMax=[]  IntegratorOutMin=[]  IntegratorOutMax=[]  FilterOutMin=[]  FilterOutMax=[]  SumOutMin=[]  SumOutMax=[]  SumI1OutMin=[]  SumI1OutMax=[]  SumI2OutMin=[]  SumI2OutMax=[]  SumI3OutMin=[]  SumI3OutMax=[]  SumDOutMin=[]  SumDOutMax=[]  SaturationOutMin=[]  SaturationOutMax=[]  IntegratorContinuousStateAttributes=''  IntegratorStateMustResolveToSignalObject=off  IntegratorRTWStateStorageClass=Auto  FilterContinuousStateAttributes=''  FilterStateMustResolveToSignalObject=off  FilterRTWStateStorageClass=Auto  DifferentiatorICPrevScaledInput=0  DifferentiatorOutMin=[]  DifferentiatorOutMax=[]
  Sum : Sum  Inputs=|+-
  Sum1 : Sum  Inputs=|+-
  Angle : Outport
  wires:
  Sum/1 -> PID Controller/1
  PID Controller/1 -> DC motor/1(Voltage)
  DC motor/1(Speed) -> Sum/2, Integrator/1
  Integrator/1 -> Angle/1, Sum1/2
  Command/1 -> Sum1/1
  Sum1/1 -> Gain/1
  Gain/1 -> Sum/1
  Constant/1 -> Integrator/2

== system PID_Dual_Robot/Joint Motor9 ==
  Command : Inport
  Constant : Constant  Value=IniJointAngle_L(2)
  DC motor : Subsystem
  Gain : Gain  Gain=2
  Integrator : Integrator  InitialConditionSource=external
  PID Controller : simulink/Continuous/PID Controller  Controller=PID  TimeDomain=Continuous-time  SampleTime=-1  IntegratorMethod=Forward Euler  FilterMethod=Forward Euler  Form=Parallel  UseFilter=on  ControllerParametersSource=internal  P=P(2)  I=I(2)  D=D(2)  N=0  InitialConditionSource=internal  InitialConditionForIntegrator=0  InitialConditionForFilter=0  ExternalReset=none  LimitOutput=off  UpperSaturationLimit=inf  LowerSaturationLimit=-inf  LinearizeAsGain=on  AntiWindupMode=none  Kb=1  TrackingMode=off  Kt=1  PParamMin=[]  PParamMax=[]  IParamMin=[]  IParamMax=[]  DParamMin=[]  DParamMax=[]  NParamMin=[]  NParamMax=[]  KbParamMin=[]  KbParamMax=[]  KtParamMin=[]  KtParamMax=[]  POutMin=[]  POutMax=[]  IOutMin=[]  IOutMax=[]  DOutMin=[]  DOutMax=[]  NOutMin=[]  NOutMax=[]  KbOutMin=[]  KbOutMax=[]  KtOutMin=[]  KtOutMax=[]  IntegratorOutMin=[]  IntegratorOutMax=[]  FilterOutMin=[]  FilterOutMax=[]  SumOutMin=[]  SumOutMax=[]  SumI1OutMin=[]  SumI1OutMax=[]  SumI2OutMin=[]  SumI2OutMax=[]  SumI3OutMin=[]  SumI3OutMax=[]  SumDOutMin=[]  SumDOutMax=[]  SaturationOutMin=[]  SaturationOutMax=[]  IntegratorContinuousStateAttributes=''  IntegratorStateMustResolveToSignalObject=off  IntegratorRTWStateStorageClass=Auto  FilterContinuousStateAttributes=''  FilterStateMustResolveToSignalObject=off  FilterRTWStateStorageClass=Auto  DifferentiatorICPrevScaledInput=0  DifferentiatorOutMin=[]  DifferentiatorOutMax=[]
  Sum : Sum  Inputs=|+-
  Sum1 : Sum  Inputs=|+-
  Angle : Outport
  wires:
  Sum/1 -> PID Controller/1
  PID Controller/1 -> DC motor/1(Voltage)
  DC motor/1(Speed) -> Sum/2, Integrator/1
  Integrator/1 -> Angle/1, Sum1/2
  Command/1 -> Sum1/1
  Sum1/1 -> Gain/1
  Gain/1 -> Sum/1
  Constant/1 -> Integrator/2

== system PID_Dual_Robot/PIDcontroller ==
  e : Inport
  D gain : Gain  Gain=TOP_D
  D scope : Scope
  Derivative : Derivative
  I gain : Gain  Gain=TOP_I
  I scope : Scope
  Integrator : Integrator
  P gain : Gain  Gain=TOP_P
  P scope : Scope
  Sum1 : Sum  Inputs=+++
  u : Outport
  wires:
  I gain/1 -> Integrator/1
  P gain/1 -> P scope/1, Sum1/1
  Integrator/1 -> I scope/1, Sum1/2
  e/1 -> D gain/1, I gain/1, P gain/1
  Sum1/1 -> u/1
  D gain/1 -> Derivative/1
  Derivative/1 -> D scope/1, Sum1/3

== system PID_Dual_Robot/PIDcontroller1 ==
  e : Inport
  D gain : Gain  Gain=TOP_D
  D scope : Scope
  Derivative : Derivative
  I gain : Gain  Gain=TOP_I
  I scope : Scope
  Integrator : Integrator
  P gain : Gain  Gain=TOP_P
  P scope : Scope
  Sum1 : Sum  Inputs=+++
  u : Outport
  wires:
  I gain/1 -> Integrator/1
  P gain/1 -> P scope/1, Sum1/1
  Integrator/1 -> I scope/1, Sum1/2
  e/1 -> D gain/1, I gain/1, P gain/1
  Sum1/1 -> u/1
  D gain/1 -> Derivative/1
  Derivative/1 -> D scope/1, Sum1/3

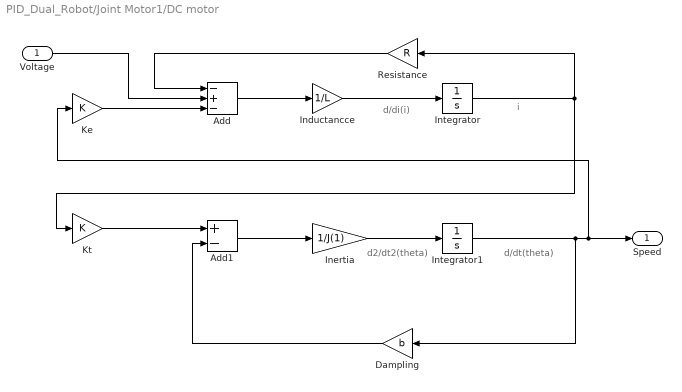
== system PID_Dual_Robot/Joint Motor1/DC motor ==
  note: d/dt(theta)
  note: d2/dt2(theta)
  note: i
  note: d/di(i)
  Voltage : Inport
  Add : Sum  Inputs=-+-
  Add1 : Sum  Inputs=+-
  Dampling : Gain  Gain=b
  Inductancce : Gain  Gain=1/L
  Inertia : Gain  Gain=1/J(1)
  Integrator : Integrator
  Integrator1 : Integrator
  Ke : Gain  Gain=K
  Kt : Gain  Gain=K
  Resistance : Gain  Gain=R
  Speed : Outport
  wires:
  Resistance/1 -> Add/1
  Add/1 -> Inductancce/1
  Inductancce/1 -> Integrator/1
  Inertia/1 -> Integrator1/1
  Kt/1 -> Add1/1
  Add1/1 -> Inertia/1
  Integrator/1 -> Kt/1, Resistance/1
  Voltage/1 -> Add/2
  Dampling/1 -> Add1/2
  Integrator1/1 -> Dampling/1, Speed/1, Ke/1
  Ke/1 -> Add/3

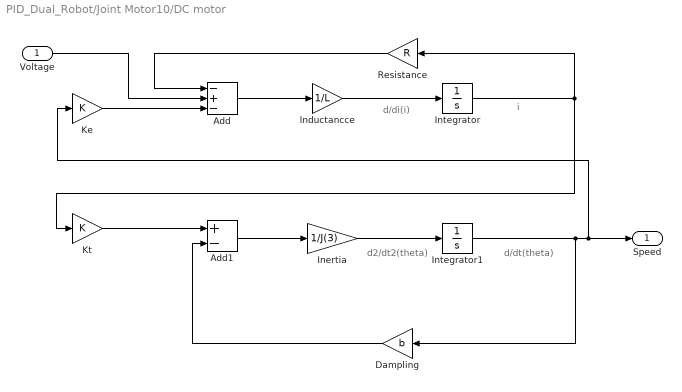
== system PID_Dual_Robot/Joint Motor10/DC motor ==
  note: d/dt(theta)
  note: d2/dt2(theta)
  note: i
  note: d/di(i)
  Voltage : Inport
  Add : Sum  Inputs=-+-
  Add1 : Sum  Inputs=+-
  Dampling : Gain  Gain=b
  Inductancce : Gain  Gain=1/L
  Inertia : Gain  Gain=1/J(3)
  Integrator : Integrator
  Integrator1 : Integrator
  Ke : Gain  Gain=K
  Kt : Gain  Gain=K
  Resistance : Gain  Gain=R
  Speed : Outport
  wires:
  Resistance/1 -> Add/1
  Add/1 -> Inductancce/1
  Inductancce/1 -> Integrator/1
  Inertia/1 -> Integrator1/1
  Kt/1 -> Add1/1
  Add1/1 -> Inertia/1
  Integrator/1 -> Kt/1, Resistance/1
  Voltage/1 -> Add/2
  Dampling/1 -> Add1/2
  Integrator1/1 -> Dampling/1, Speed/1, Ke/1
  Ke/1 -> Add/3

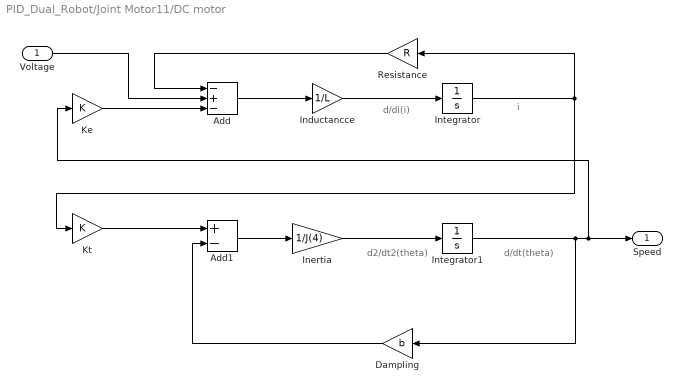
== system PID_Dual_Robot/Joint Motor11/DC motor ==
  note: d/dt(theta)
  note: d2/dt2(theta)
  note: i
  note: d/di(i)
  Voltage : Inport
  Add : Sum  Inputs=-+-
  Add1 : Sum  Inputs=+-
  Dampling : Gain  Gain=b
  Inductancce : Gain  Gain=1/L
  Inertia : Gain  Gain=1/J(4)
  Integrator : Integrator
  Integrator1 : Integrator
  Ke : Gain  Gain=K
  Kt : Gain  Gain=K
  Resistance : Gain  Gain=R
  Speed : Outport
  wires:
  Resistance/1 -> Add/1
  Add/1 -> Inductancce/1
  Inductancce/1 -> Integrator/1
  Inertia/1 -> Integrator1/1
  Kt/1 -> Add1/1
  Add1/1 -> Inertia/1
  Integrator/1 -> Kt/1, Resistance/1
  Voltage/1 -> Add/2
  Dampling/1 -> Add1/2
  Integrator1/1 -> Dampling/1, Speed/1, Ke/1
  Ke/1 -> Add/3

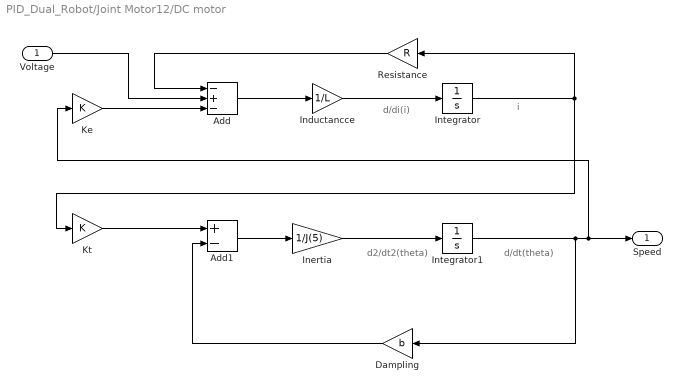
== system PID_Dual_Robot/Joint Motor12/DC motor ==
  note: d/dt(theta)
  note: d2/dt2(theta)
  note: i
  note: d/di(i)
  Voltage : Inport
  Add : Sum  Inputs=-+-
  Add1 : Sum  Inputs=+-
  Dampling : Gain  Gain=b
  Inductancce : Gain  Gain=1/L
  Inertia : Gain  Gain=1/J(5)
  Integrator : Integrator
  Integrator1 : Integrator
  Ke : Gain  Gain=K
  Kt : Gain  Gain=K
  Resistance : Gain  Gain=R
  Speed : Outport
  wires:
  Resistance/1 -> Add/1
  Add/1 -> Inductancce/1
  Inductancce/1 -> Integrator/1
  Inertia/1 -> Integrator1/1
  Kt/1 -> Add1/1
  Add1/1 -> Inertia/1
  Integrator/1 -> Kt/1, Resistance/1
  Voltage/1 -> Add/2
  Dampling/1 -> Add1/2
  Integrator1/1 -> Dampling/1, Speed/1, Ke/1
  Ke/1 -> Add/3

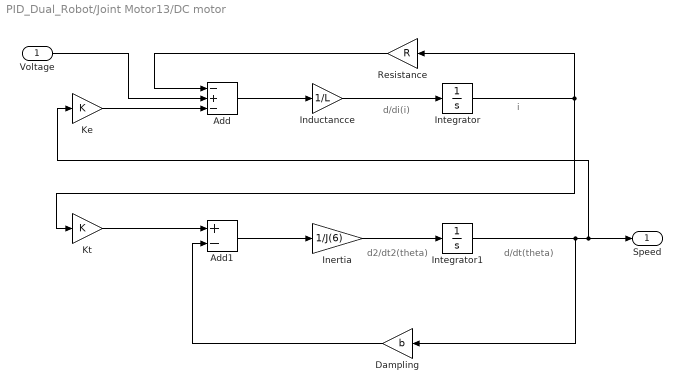
== system PID_Dual_Robot/Joint Motor13/DC motor ==
  note: d/dt(theta)
  note: d2/dt2(theta)
  note: i
  note: d/di(i)
  Voltage : Inport
  Add : Sum  Inputs=-+-
  Add1 : Sum  Inputs=+-
  Dampling : Gain  Gain=b
  Inductancce : Gain  Gain=1/L
  Inertia : Gain  Gain=1/J(6)
  Integrator : Integrator
  Integrator1 : Integrator
  Ke : Gain  Gain=K
  Kt : Gain  Gain=K
  Resistance : Gain  Gain=R
  Speed : Outport
  wires:
  Resistance/1 -> Add/1
  Add/1 -> Inductancce/1
  Inductancce/1 -> Integrator/1
  Inertia/1 -> Integrator1/1
  Kt/1 -> Add1/1
  Add1/1 -> Inertia/1
  Integrator/1 -> Kt/1, Resistance/1
  Voltage/1 -> Add/2
  Dampling/1 -> Add1/2
  Integrator1/1 -> Dampling/1, Speed/1, Ke/1
  Ke/1 -> Add/3

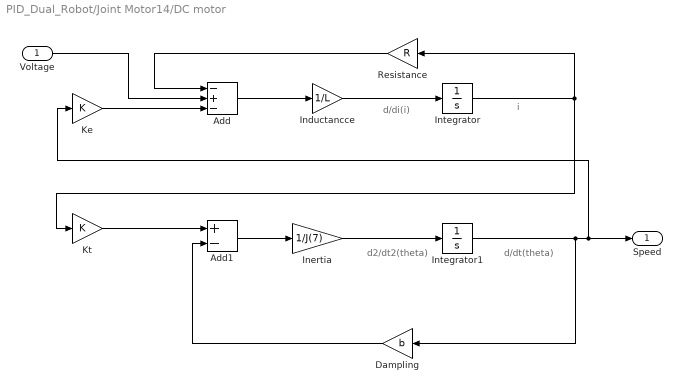
== system PID_Dual_Robot/Joint Motor14/DC motor ==
  note: d/dt(theta)
  note: d2/dt2(theta)
  note: i
  note: d/di(i)
  Voltage : Inport
  Add : Sum  Inputs=-+-
  Add1 : Sum  Inputs=+-
  Dampling : Gain  Gain=b
  Inductancce : Gain  Gain=1/L
  Inertia : Gain  Gain=1/J(7)
  Integrator : Integrator
  Integrator1 : Integrator
  Ke : Gain  Gain=K
  Kt : Gain  Gain=K
  Resistance : Gain  Gain=R
  Speed : Outport
  wires:
  Resistance/1 -> Add/1
  Add/1 -> Inductancce/1
  Inductancce/1 -> Integrator/1
  Inertia/1 -> Integrator1/1
  Kt/1 -> Add1/1
  Add1/1 -> Inertia/1
  Integrator/1 -> Kt/1, Resistance/1
  Voltage/1 -> Add/2
  Dampling/1 -> Add1/2
  Integrator1/1 -> Dampling/1, Speed/1, Ke/1
  Ke/1 -> Add/3

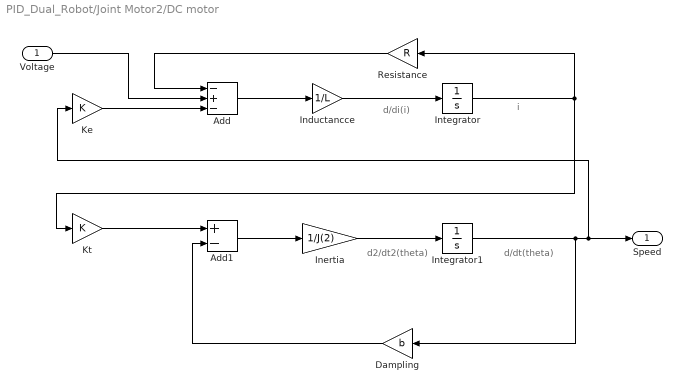
== system PID_Dual_Robot/Joint Motor2/DC motor ==
  note: d/dt(theta)
  note: d2/dt2(theta)
  note: i
  note: d/di(i)
  Voltage : Inport
  Add : Sum  Inputs=-+-
  Add1 : Sum  Inputs=+-
  Dampling : Gain  Gain=b
  Inductancce : Gain  Gain=1/L
  Inertia : Gain  Gain=1/J(2)
  Integrator : Integrator
  Integrator1 : Integrator
  Ke : Gain  Gain=K
  Kt : Gain  Gain=K
  Resistance : Gain  Gain=R
  Speed : Outport
  wires:
  Resistance/1 -> Add/1
  Add/1 -> Inductancce/1
  Inductancce/1 -> Integrator/1
  Inertia/1 -> Integrator1/1
  Kt/1 -> Add1/1
  Add1/1 -> Inertia/1
  Integrator/1 -> Kt/1, Resistance/1
  Voltage/1 -> Add/2
  Dampling/1 -> Add1/2
  Integrator1/1 -> Dampling/1, Speed/1, Ke/1
  Ke/1 -> Add/3

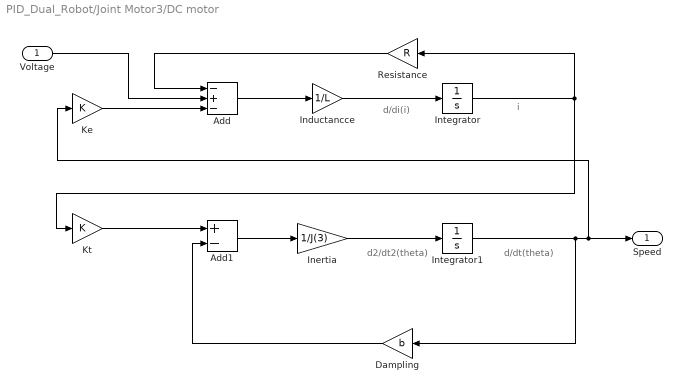
== system PID_Dual_Robot/Joint Motor3/DC motor ==
  note: d/dt(theta)
  note: d2/dt2(theta)
  note: i
  note: d/di(i)
  Voltage : Inport
  Add : Sum  Inputs=-+-
  Add1 : Sum  Inputs=+-
  Dampling : Gain  Gain=b
  Inductancce : Gain  Gain=1/L
  Inertia : Gain  Gain=1/J(3)
  Integrator : Integrator
  Integrator1 : Integrator
  Ke : Gain  Gain=K
  Kt : Gain  Gain=K
  Resistance : Gain  Gain=R
  Speed : Outport
  wires:
  Resistance/1 -> Add/1
  Add/1 -> Inductancce/1
  Inductancce/1 -> Integrator/1
  Inertia/1 -> Integrator1/1
  Kt/1 -> Add1/1
  Add1/1 -> Inertia/1
  Integrator/1 -> Kt/1, Resistance/1
  Voltage/1 -> Add/2
  Dampling/1 -> Add1/2
  Integrator1/1 -> Dampling/1, Speed/1, Ke/1
  Ke/1 -> Add/3

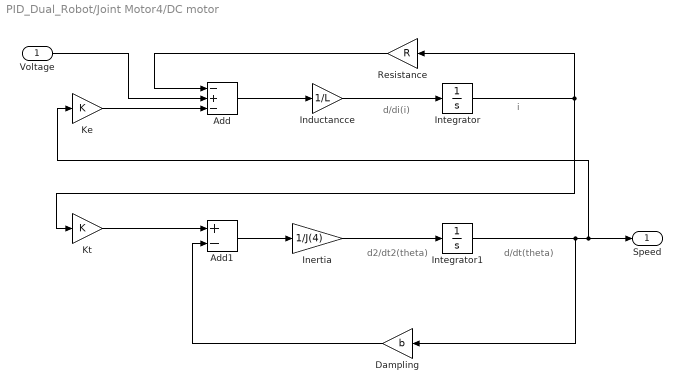
== system PID_Dual_Robot/Joint Motor4/DC motor ==
  note: d/dt(theta)
  note: d2/dt2(theta)
  note: i
  note: d/di(i)
  Voltage : Inport
  Add : Sum  Inputs=-+-
  Add1 : Sum  Inputs=+-
  Dampling : Gain  Gain=b
  Inductancce : Gain  Gain=1/L
  Inertia : Gain  Gain=1/J(4)
  Integrator : Integrator
  Integrator1 : Integrator
  Ke : Gain  Gain=K
  Kt : Gain  Gain=K
  Resistance : Gain  Gain=R
  Speed : Outport
  wires:
  Resistance/1 -> Add/1
  Add/1 -> Inductancce/1
  Inductancce/1 -> Integrator/1
  Inertia/1 -> Integrator1/1
  Kt/1 -> Add1/1
  Add1/1 -> Inertia/1
  Integrator/1 -> Kt/1, Resistance/1
  Voltage/1 -> Add/2
  Dampling/1 -> Add1/2
  Integrator1/1 -> Dampling/1, Speed/1, Ke/1
  Ke/1 -> Add/3

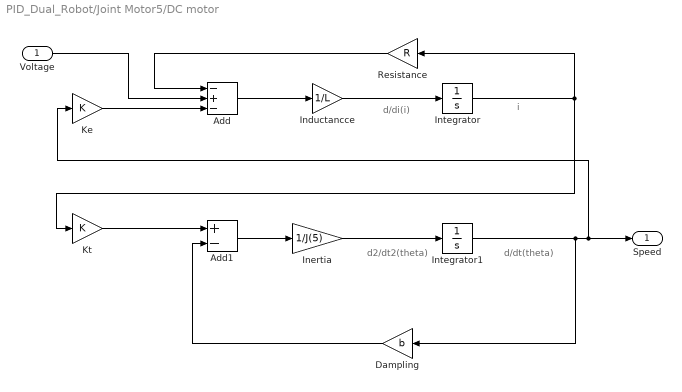
== system PID_Dual_Robot/Joint Motor5/DC motor ==
  note: d/dt(theta)
  note: d2/dt2(theta)
  note: i
  note: d/di(i)
  Voltage : Inport
  Add : Sum  Inputs=-+-
  Add1 : Sum  Inputs=+-
  Dampling : Gain  Gain=b
  Inductancce : Gain  Gain=1/L
  Inertia : Gain  Gain=1/J(5)
  Integrator : Integrator
  Integrator1 : Integrator
  Ke : Gain  Gain=K
  Kt : Gain  Gain=K
  Resistance : Gain  Gain=R
  Speed : Outport
  wires:
  Resistance/1 -> Add/1
  Add/1 -> Inductancce/1
  Inductancce/1 -> Integrator/1
  Inertia/1 -> Integrator1/1
  Kt/1 -> Add1/1
  Add1/1 -> Inertia/1
  Integrator/1 -> Kt/1, Resistance/1
  Voltage/1 -> Add/2
  Dampling/1 -> Add1/2
  Integrator1/1 -> Dampling/1, Speed/1, Ke/1
  Ke/1 -> Add/3

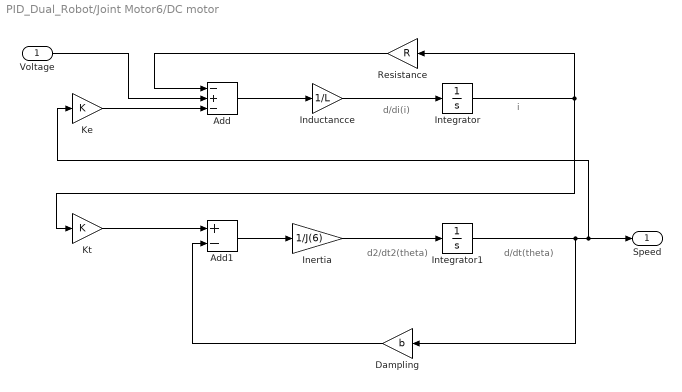
== system PID_Dual_Robot/Joint Motor6/DC motor ==
  note: d/dt(theta)
  note: d2/dt2(theta)
  note: i
  note: d/di(i)
  Voltage : Inport
  Add : Sum  Inputs=-+-
  Add1 : Sum  Inputs=+-
  Dampling : Gain  Gain=b
  Inductancce : Gain  Gain=1/L
  Inertia : Gain  Gain=1/J(6)
  Integrator : Integrator
  Integrator1 : Integrator
  Ke : Gain  Gain=K
  Kt : Gain  Gain=K
  Resistance : Gain  Gain=R
  Speed : Outport
  wires:
  Resistance/1 -> Add/1
  Add/1 -> Inductancce/1
  Inductancce/1 -> Integrator/1
  Inertia/1 -> Integrator1/1
  Kt/1 -> Add1/1
  Add1/1 -> Inertia/1
  Integrator/1 -> Kt/1, Resistance/1
  Voltage/1 -> Add/2
  Dampling/1 -> Add1/2
  Integrator1/1 -> Dampling/1, Speed/1, Ke/1
  Ke/1 -> Add/3

== system PID_Dual_Robot/Joint Motor7/DC motor ==
  note: d/dt(theta)
  note: d2/dt2(theta)
  note: i
  note: d/di(i)
  Voltage : Inport
  Add : Sum  Inputs=-+-
  Add1 : Sum  Inputs=+-
  Dampling : Gain  Gain=b
  Inductancce : Gain  Gain=1/L
  Inertia : Gain  Gain=1/J(7)
  Integrator : Integrator
  Integrator1 : Integrator
  Ke : Gain  Gain=K
  Kt : Gain  Gain=K
  Resistance : Gain  Gain=R
  Speed : Outport
  wires:
  Resistance/1 -> Add/1
  Add/1 -> Inductancce/1
  Inductancce/1 -> Integrator/1
  Inertia/1 -> Integrator1/1
  Kt/1 -> Add1/1
  Add1/1 -> Inertia/1
  Integrator/1 -> Kt/1, Resistance/1
  Voltage/1 -> Add/2
  Dampling/1 -> Add1/2
  Integrator1/1 -> Dampling/1, Speed/1, Ke/1
  Ke/1 -> Add/3

== system PID_Dual_Robot/Joint Motor8/DC motor ==
  note: d/dt(theta)
  note: d2/dt2(theta)
  note: i
  note: d/di(i)
  Voltage : Inport
  Add : Sum  Inputs=-+-
  Add1 : Sum  Inputs=+-
  Dampling : Gain  Gain=b
  Inductancce : Gain  Gain=1/L
  Inertia : Gain  Gain=1/J(1)
  Integrator : Integrator
  Integrator1 : Integrator
  Ke : Gain  Gain=K
  Kt : Gain  Gain=K
  Resistance : Gain  Gain=R
  Speed : Outport
  wires:
  Resistance/1 -> Add/1
  Add/1 -> Inductancce/1
  Inductancce/1 -> Integrator/1
  Inertia/1 -> Integrator1/1
  Kt/1 -> Add1/1
  Add1/1 -> Inertia/1
  Integrator/1 -> Kt/1, Resistance/1
  Voltage/1 -> Add/2
  Dampling/1 -> Add1/2
  Integrator1/1 -> Dampling/1, Speed/1, Ke/1
  Ke/1 -> Add/3

== system PID_Dual_Robot/Joint Motor9/DC motor ==
  note: d/dt(theta)
  note: d2/dt2(theta)
  note: i
  note: d/di(i)
  Voltage : Inport
  Add : Sum  Inputs=-+-
  Add1 : Sum  Inputs=+-
  Dampling : Gain  Gain=b
  Inductancce : Gain  Gain=1/L
  Inertia : Gain  Gain=1/J(2)
  Integrator : Integrator
  Integrator1 : Integrator
  Ke : Gain  Gain=K
  Kt : Gain  Gain=K
  Resistance : Gain  Gain=R
  Speed : Outport
  wires:
  Resistance/1 -> Add/1
  Add/1 -> Inductancce/1
  Inductancce/1 -> Integrator/1
  Inertia/1 -> Integrator1/1
  Kt/1 -> Add1/1
  Add1/1 -> Inertia/1
  Integrator/1 -> Kt/1, Resistance/1
  Voltage/1 -> Add/2
  Dampling/1 -> Add1/2
  Integrator1/1 -> Dampling/1, Speed/1, Ke/1
  Ke/1 -> Add/3
